simulink model "FOC_DQ0_EMR"  (R2022b)
settings: Solver=ode23s  StartTime=0.0  StopTime=50  MaxStep=1e-3
values from neighbouring files (symbols this model uses):
  battery = struct()    [FOC_DQ0_parameters.m]
  car = struct()    [FOC_DQ0_parameters.m]
  inv = struct()    [FOC_DQ0_parameters.m]
  motor = struct()    [FOC_DQ0_parameters.m]
libraries: simulink_extras x7, simulink x6, cstblocks x1
settings Model: Creator=dwegg  LastModifiedBy=dwegg
settings SolverCC: MaxConsecutiveZCs=auto  AlgebraicLoopSolver=TrustRegion
settings OptimizationCC: OptimizeBlockIOStorage=off  OptimizeDataStoreBuffers=off  BusAssignmentInplaceUpdate=off
settings DebuggingCC: UnconnectedInputMsg=warning  UnconnectedOutputMsg=warning  UnconnectedLineMsg=warning  UniqueDataStoreMsg=error  SFUnexpectedBacktrackingDiag=warning  SFNoUnconditionalDefaultTransitionDiag=warning  SFMachineParentedDataDiag=warning
settings ModelReferenceCC: EnableRefExpFcnMdlSchedulingChecks=on
settings RTWCC: GenCodeOnly=on  GenerateReport=on  BuildConfiguration=Debug  LaunchReport=on  DLArmComputeVersion=19.05
settings CodeAppCC: ForceParamTrailComments=on  MATLABSourceComments=on  EnableCustomComments=on
settings GRTTargetCC: CombineSignalStateStructs=on  SupportVariableSizeSignals=on  MultiInstanceErrorCode=Warning

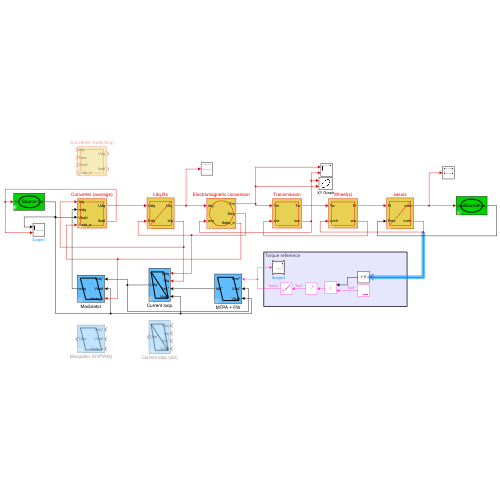
[thumbnail: Simulink's stored preview of the top-level diagram]
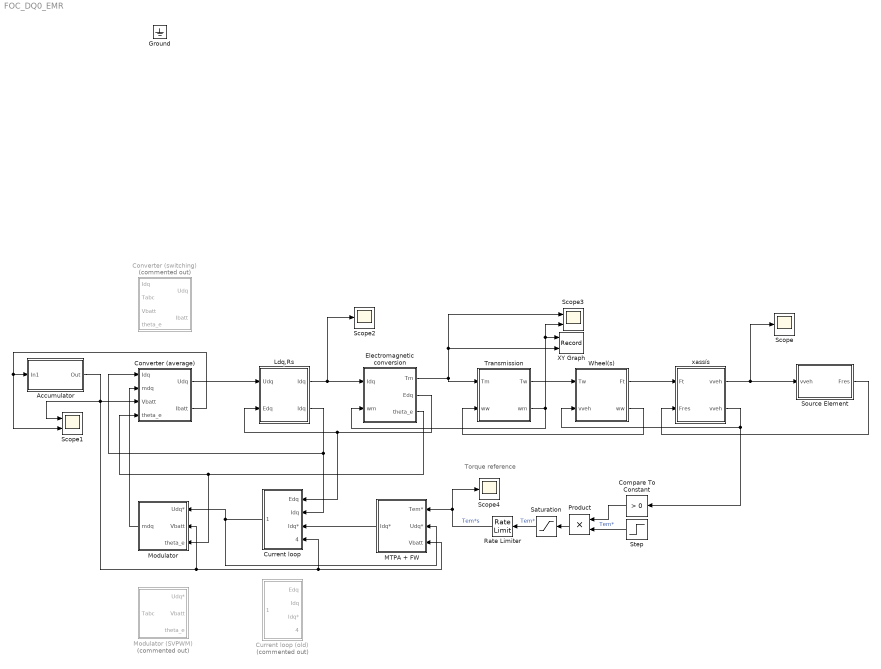
== system FOC_DQ0_EMR ==
  note: Torque reference
  Accumulator : Subsystem  AncestorBlock=simulink/REM/SE
      settings: LibrarySourceBlock=simulink/REM/SE
      mask Display:
      | plot(0,0,100,100, 1.2*[50,57.68,60.77,63.08,64.97,66.58,68,69.26,70.4, 	71.42,72.36,78.28,80,78.28,72.36,71.42,70.4, 	69.26,68,66.58,64.97,63.08,60.77,57.68,50,42.32, 	39.23,36.92,35.03,33.42,32,30.74,29.6,28.58, 	27.64,21.72,20,21.72,27.64,28.58,29.6,30.74,32, 	33.42,35.03,36.92,39.23,42.32,50]-10, 1.2*[20,21,22,23,24,25,26,27,28,29,30,40,50,60,70,71,72, 	73,74,75,76,77,78,79,80,79,78,77,76,75,74,73,72, 	71,70,60,50,40,30,29,28,27,26,25,24,23,22,21,20]-10)
      | disp('Source')
  Compare To Constant : simulink/Logic and Bit Operations/Compare To Constant  relop=>  const=0  OutDataTypeStr=boolean
  Converter (average) : Subsystem  AncestorBlock=simulink/REM/EC Elec  mask(Hacheur){}
      settings: LibrarySourceBlock=simulink/REM/EC Elec
      mask Display: plot(0,0,100,100,[10,10,90,90,10],[90,10,10,90,90])
  Converter (switching) : Subsystem  Commented=on  AncestorBlock=simulink/REM/EC Elec  mask(Hacheur){}
      settings: LibrarySourceBlock=simulink/REM/EC Elec
      mask Display: plot(0,0,100,100,[10,10,90,90,10],[90,10,10,90,90])
  Current loop : Subsystem  AncestorBlock=simulink/SMC/Asservissement Correcteur IP
      settings: LibrarySourceBlock=|
      | simulink/SMC/Asservissement
      | Correcteur IP
      mask Display: plot(0,0,100,100, [10,30,90,70,10,90],[90,10,10,90,90,10])
  Current loop (old) : Subsystem  Commented=on  AncestorBlock=simulink/SMC/Asservissement Correcteur IP
      settings: LibrarySourceBlock=|
      | simulink/SMC/Asservissement
      | Correcteur IP
      mask Display: plot(0,0,100,100, [10,30,90,70,10,90],[90,10,10,90,90,10])
  Electromagnetic conversion : Subsystem  AncestorBlock=simulink/REM/EC EM
      settings: LibrarySourceBlock=simulink/REM/EC EM
      mask Display: plot(0,0,100,100, 1.4*[50,57.68,60.77,63.08,64.97,66.58,68,69.26,70.4, 	71.42,72.36,78.28,80,78.28,72.36,71.42,70.4, 	69.26,68,66.58,64.97,63.08,60.77,57.68,50,42.32, 	39.23,36.92,35.03,33.42,32,30.74,29.6,28.58, 	27.64,21.72,20,21.72,27.64,28.58,29.6,30.74,32, 	33.42,35.03,36.92,39.23,42.32,50]-20, 1.4*[20,21,22,23,24,25,26,27,28,29,30,40,50,60,70,71,72, 	73,74,75,76,77,78,79,80,79,78,77,76,75,74,73,72, 	71,70,60,50,40,30,29,28,27,26,25,24,23,22,21,20]-20)
  Ldq,Rs : Subsystem  AncestorBlock=simulink/REM/EA  mask(CM){}
      settings: LibrarySourceBlock=simulink/REM/EA
      mask Display: plot(0,0,100,100,[10,10,90,90,10],[90,10,10,90,90], [10,90],[10,90])
  MTPA + FW : Subsystem  AncestorBlock=simulink/SMC/Inversion EC avec mesure
      settings: LibrarySourceBlock=|
      | simulink/SMC/Inversion EC
      | avec mesure
      mask Display: plot(0,0,100,100,[10,30,90,70,10],[90,10,10,90,90])
  Modulator : Subsystem  AncestorBlock=simulink/SMC/Inversion EC avec mesure
      settings: LibrarySourceBlock=|
      | simulink/SMC/Inversion EC
      | avec mesure
      mask Display: plot(0,0,100,100,[10,30,90,70,10],[90,10,10,90,90])
  Modulator (SVPWM) : Subsystem  Commented=on  AncestorBlock=simulink/SMC/Inversion EC avec mesure
      settings: LibrarySourceBlock=|
      | simulink/SMC/Inversion EC
      | avec mesure
      mask Display: plot(0,0,100,100,[10,30,90,70,10],[90,10,10,90,90])
  Product : Product
  Rate Limiter : RateLimiter  RisingSlewLimit=motor.Te_max*10  FallingSlewLimit=-motor.Te_max*10  SampleTimeMode=inherited
  Saturation : Saturate  UpperLimit=motor.Te_max*1.2  LowerLimit=-motor.Te_max*1.2
  Scope : Scope
  Scope1 : Scope  NumInputPorts=2
  Scope2 : Scope
  Scope3 : Scope  NumInputPorts=2
  Scope4 : Scope
  Source Element : Subsystem  AncestorBlock=simulink/REM/SE
      settings: LibrarySourceBlock=simulink/REM/SE
      mask Display:
      | plot(0,0,100,100, 1.2*[50,57.68,60.77,63.08,64.97,66.58,68,69.26,70.4, 	71.42,72.36,78.28,80,78.28,72.36,71.42,70.4, 	69.26,68,66.58,64.97,63.08,60.77,57.68,50,42.32, 	39.23,36.92,35.03,33.42,32,30.74,29.6,28.58, 	27.64,21.72,20,21.72,27.64,28.58,29.6,30.74,32, 	33.42,35.03,36.92,39.23,42.32,50]-10, 1.2*[20,21,22,23,24,25,26,27,28,29,30,40,50,60,70,71,72, 	73,74,75,76,77,78,79,80,79,78,77,76,75,74,73,72, 	71,70,60,50,40,30,29,28,27,26,25,24,23,22,21,20]-10)
      | disp('Source')
  Step : Step  Time=25  Before=150  After=-150  SampleTime=0
  Transmission : Subsystem  AncestorBlock=simulink/REM/EC Elec  mask(Hacheur){}
      settings: LibrarySourceBlock=simulink/REM/EC Elec
      mask Display: plot(0,0,100,100,[10,10,90,90,10],[90,10,10,90,90])
  Wheel(s) : Subsystem  AncestorBlock=simulink/REM/EC Elec  mask(Hacheur){}
      settings: LibrarySourceBlock=simulink/REM/EC Elec
      mask Display: plot(0,0,100,100,[10,10,90,90,10],[90,10,10,90,90])
  XY Graph : Record  FileSettingsInternal="{\"entries\":[{\"content\":{\"excelSettings\":{\"content\":{},\"type\":\"Streamout.ExcelSettings\"}},\"type\":\"Streamout.FileSettingStorage\",\"uuid\":\"4b251279-da9d-4be6-a887-ea3e78efb50d\"}],\"packageUris\":[\"http://schema.mathworks.com/mf0/streamout_blocks/R2020a\"],\"version\":\"1.0\"}"  Layout=[1 1]  SignalsInternal="{\"entries\":[{\"content\":{\"signals\":[{\"content\":{\"blockPath\":[\"FOC_DQ0_EMR/XY Graph\"],\"channel\":[],\"dimensions\":[1],\"domain\":\"FOC_DQ0_EMR/XY Graph\",\"lineColor\":\"#a2142f\",\"plots\":[1],\"port\":1,\"sid\":[\"\"],\"signalID\":135004,\"signalName\":\"Transmission:2\"},\"type\":\"RecordBlkView.Signal\",\"uuid\":\"7b1c68ec-b94b-4dc4-ac7b-7f2c86aeb692\"},{\"content\":{\"blockPath\":[\"FOC_DQ0_EMR/XY Graph\"],\"channel\":[],\"dimensions\":[1],\"domain\":\"FOC_DQ0_EMR/XY Graph\",\"lineColor\":\"#139fff\",\"plots\":[1],\"port\":2,\"sid\":[\"\"],\"signalID\":135008,\"signalName\":\"Electromagnetic conversion:1\"},\"type\":\"RecordBlkView.Signal\",\"uuid\":\"55ce29f7-d8dd-4043-829a-ad02527bc7f8\"}]},\"type\":\"RecordBlkView.InputSignals\",\"uuid\":\"8a0fc05b-648f-47b4-bd4d-9f4339ba604a\"}],\"packageUris\":[\"http://schema.mathworks.com/mf0/streamout_blocks/R2020a\"],\"version\":\"1.0\"}"  VisualizationBindings="{\"xyplotplugin\":{\"info\":[{\"series\":[{\"bindingParametersList\":[{\"parameter\":\"X-Axis\",\"signalID\":135004,\"signalName\":\"Transmission:2\"},{\"parameter\":\"Y-Axis\",\"signalID\":135008,\"signalName\":\"Electromagnetic conversion:1\"}],\"seriesID\":21416}],\"subplotID\":1}]}}"  CompatibilityTag=XY
  xassís : Subsystem  AncestorBlock=simulink/REM/EA  mask(CM){}
      settings: LibrarySourceBlock=simulink/REM/EA
      mask Display: plot(0,0,100,100,[10,10,90,90,10],[90,10,10,90,90], [10,90],[10,90])
  Ground : Ground  IOType=siggen
  wires:
  Accumulator/1(Out) -> Scope1/1, Converter (average)/3(Vbatt), Modulator/2(Vbatt), Current loop/4(Vbatt), MTPA + FW/3(Vbatt)
  Step/1 -> Product/2  "Tem*"
  Saturation/1 -> Rate Limiter/1  "Tem*"
  Electromagnetic conversion/2(Edq) -> Current loop/1(Edq), Ldq,Rs/2(Edq)
  Converter (average)/1(Udq) -> Ldq,Rs/1(Udq)
  Ldq,Rs/2(Idq) -> Current loop/2(Idq), Converter (average)/1(Idq)
  Converter (average)/2(Ibatt) -> Scope1/2, Accumulator/1(In1)
  Electromagnetic conversion/1(Tm) -> Transmission/1(Tm), XY Graph/2, Scope3/1
  Transmission/2(wm) -> XY Graph/1, Scope3/2, Electromagnetic conversion/2(wm)
  Transmission/1(Tw) -> Wheel(s)/1(Tw)
  Wheel(s)/2(ww) -> Transmission/2(ww)
  Current loop/1(Udq*) -> Modulator/1(Udq*), MTPA + FW/2(Udq*)
  MTPA + FW/1(Idq*) -> Current loop/3(Idq*)
  Wheel(s)/1(Ft) -> xassís/1(Ft)
  xassís/1(vveh) -> Scope/1, Source Element/1(vveh)
  Source Element/1(Fres) -> xassís/2(Fres)
  Ldq,Rs/1("Idq ") -> Scope2/1, Electromagnetic conversion/1(Idq)
  Rate Limiter/1 -> Scope4/1, MTPA + FW/1(Tem*)  "Tem*s"
  Electromagnetic conversion/3(theta_e) -> Converter (average)/4(theta_e), Modulator/3(theta_e)
  Modulator/1(mdq) -> Converter (average)/2(mdq)
  Product/1 -> Saturation/1
  Compare To Constant/1 -> Product/1
  xassís/2("vveh ") -> Compare To Constant/1, Wheel(s)/2(vveh)

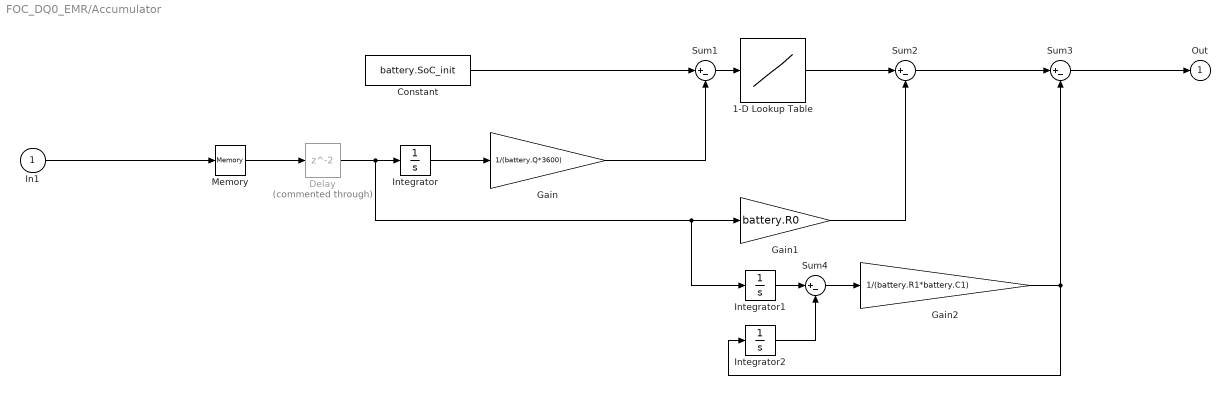
== system FOC_DQ0_EMR/Accumulator ==
  In1 : Inport
  1-D Lookup Table : Lookup_n-D  NumberOfTableDimensions=1  BreakpointsForDimension1=battery.SoC/100  Table=battery.OCV  InternalRulePriority=Speed  RndMeth=Simplest
  Constant : Constant  Value=battery.SoC_init
  Delay : Delay  Commented=through
  Gain : Gain  Gain=1/(battery.Q*3600)
  Gain1 : Gain  Gain=battery.R0
  Gain2 : Gain  Gain=1/(battery.R1*battery.C1)
  Integrator : Integrator
  Integrator1 : Integrator
  Integrator2 : Integrator
  Memory : Memory
  Sum{1..4} (4 alike) : Sum  Inputs=|+-
  Out : Outport  InitialOutput=0
  wires:
  Sum3/1 -> Out/1
  Integrator/1 -> Gain/1
  Constant/1 -> Sum1/1
  Sum1/1 -> 1-D Lookup Table/1
  Gain/1 -> Sum1/2
  1-D Lookup Table/1 -> Sum2/1
  Gain1/1 -> Sum2/2
  Sum2/1 -> Sum3/1
  Integrator1/1 -> Sum4/1
  Integrator2/1 -> Sum4/2
  Sum4/1 -> Gain2/1
  Gain2/1 -> Integrator2/1, Sum3/2
  Delay/1 -> Integrator1/1, Gain1/1, Integrator/1
  In1/1 -> Memory/1
  Memory/1 -> Delay/1

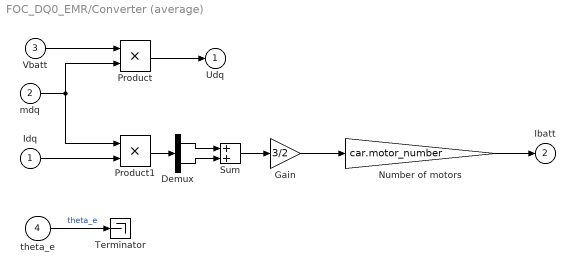
== system FOC_DQ0_EMR/Converter (average) ==
  Idq : Inport
  mdq : Inport  Port=2
  Vbatt : Inport  Port=3
  theta_e : Inport  Port=4
  Demux : Demux  Outputs=2
  Gain : Gain  Gain=3/2
  Number of motors : Gain  Gain=car.motor_number
  Product : Product
  Product1 : Product
  Sum : Sum
  Terminator : Terminator
  Udq : Outport  InitialOutput=0  VectorParamsAs1DForOutWhenUnconnected=off
  Ibatt : Outport  Port=2  InitialOutput=0  VectorParamsAs1DForOutWhenUnconnected=off
  wires:
  Vbatt/1 -> Product/1
  mdq/1 -> Product1/1, Product/2
  Product/1 -> Udq/1
  Product1/1 -> Demux/1
  Demux/1 -> Sum/1
  Demux/2 -> Sum/2
  Sum/1 -> Gain/1
  Gain/1 -> Number of motors/1
  Idq/1 -> Product1/2
  Number of motors/1 -> Ibatt/1
  theta_e/1 -> Terminator/1  "theta_e"

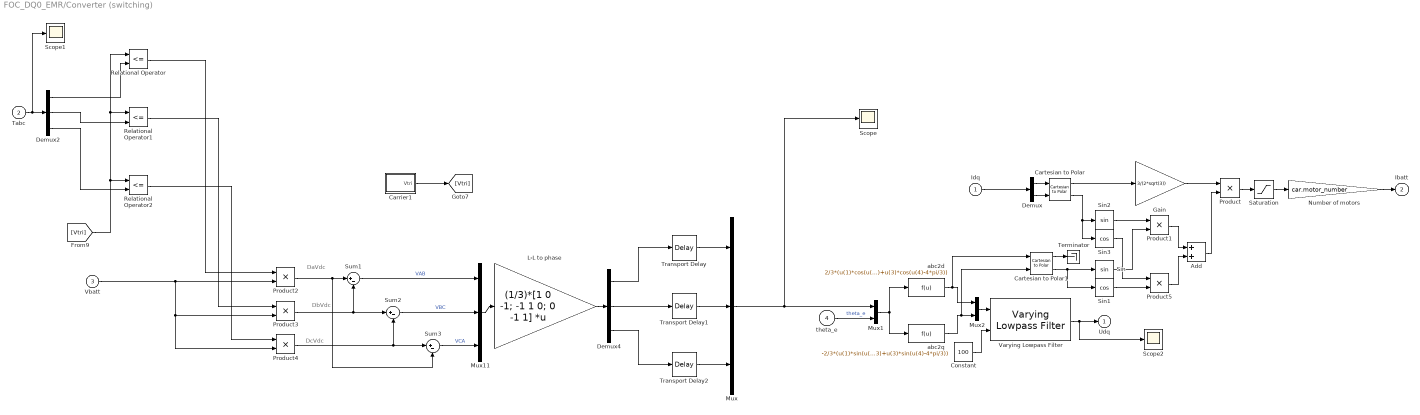
== system FOC_DQ0_EMR/Converter (switching) ==
  note: DaVdc
  note: DbVdc
  note: DcVdc
  Idq : Inport
  Tabc : Inport  Port=2
  Vbatt : Inport  Port=3
  theta_e : Inport  Port=4
  Add : Sum
  Carrier1 : Subsystem  mask{fsw=inv.fsw}
      mask prompts: fsw "switching frequency"
      mask init:
      | fsw2=fsw*2;
      | x=[0 1/4 3/4 1];
      | y=[0 -1     1    0];
      mask Display: plot([x  x+1 ],[y y])
  Cartesian to Polar : simulink_extras/Transformations/Cartesian to Polar
  Cartesian to Polar1 : simulink_extras/Transformations/Cartesian to Polar
  Constant : Constant  Value=100
  Demux : Demux  Outputs=2
  Demux2 : Demux  Outputs=3
  Demux4 : Demux  Outputs=3
  Gain : Gain  Gain=3/(2*sqrt(3))
  "L-L to phase " : Gain  Gain=(1/3)*[1 0 -1; -1 1 0; 0 -1 1]  Multiplication=Matrix(K*u)
  Mux : Mux  Inputs=3
  Mux1 : Mux  Inputs=2
  Mux11 : Mux  Inputs=3
  Mux2 : Mux  Inputs=2
  Number of motors : Gain  Gain=car.motor_number
  Product{,1..5} (6 alike) : Product
  Relational Operator : RelationalOperator  Operator=<=  OutDataTypeStr=boolean  ZeroCross=off  RndMeth=Simplest  InputSameDT=off
  Relational Operator1 : RelationalOperator  Operator=<=  OutDataTypeStr=boolean  ZeroCross=off  RndMeth=Simplest  InputSameDT=off
  Relational Operator2 : RelationalOperator  Operator=<=  OutDataTypeStr=boolean  ZeroCross=off  RndMeth=Simplest  InputSameDT=off
  Saturation : Saturate  UpperLimit=300  LowerLimit=-300
  Scope : Scope
  Scope1 : Scope
  Scope2 : Scope
  Sin : Trigonometry
  Sin1 : Trigonometry  Operator=cos
  Sin2 : Trigonometry
  Sin3 : Trigonometry  Operator=cos
  Sum1 : Sum  Inputs=|+-
  Sum2 : Sum  Inputs=|+-
  Sum3 : Sum  Inputs=|+-
  Terminator : Terminator
  Transport Delay : TransportDelay  DelayTime=inv.Tsw/2
  Transport Delay1 : TransportDelay  DelayTime=inv.Tsw/2
  Transport Delay2 : TransportDelay  DelayTime=inv.Tsw/2
  Varying Lowpass Filter : cstblocks/Linear Parameter Varying/Varying Lowpass Filter  N=1
  abc2d : Fcn  Expr=2/3*(u(1)*cos(u(4))+u(2)*cos(u(4)-2*pi/3)+u(3)*cos(u(4)-4*pi/3))
  abc2q : Fcn  Expr=-2/3*(u(1)*sin(u(4))+u(2)*sin(u(4)-2*pi/3)+u(3)*sin(u(4)-4*pi/3))
  Udq : Outport  InitialOutput=0  VectorParamsAs1DForOutWhenUnconnected=off
  Ibatt : Outport  Port=2  InitialOutput=0  VectorParamsAs1DForOutWhenUnconnected=off
  wires:
  Product/1 -> Saturation/1
  Idq/1 -> Demux/1
  Number of motors/1 -> Ibatt/1
  Demux2/1 -> Relational Operator/2
  Tabc/1 -> Scope1/1, Demux2/1
  Transport Delay2/1 -> Mux/3
  Demux4/1 -> Transport Delay/1
  Transport Delay1/1 -> Mux/2
  Relational Operator1/1 -> Product3/1
  Sum2/1 -> Mux11/2  "VBC"
  Demux4/2 -> Transport Delay1/1
  Sum1/1 -> Mux11/1  "VAB"
  Vbatt/1 -> Product4/2, Product3/2, Product2/2
  Demux4/3 -> Transport Delay2/1
  Product4/1 -> Sum3/1, Sum2/2
  Relational Operator/1 -> Product2/1
  Transport Delay/1 -> Mux/1
  "L-L to phase "/1 -> Demux4/1
  Demux2/2 -> Relational Operator1/2
  Relational Operator2/1 -> Product4/1
  Product3/1 -> Sum2/1, Sum1/2
  Carrier1/1(Vtri) -> [Vtri]
  Mux11/1 -> "L-L to phase "/1
  Demux2/3 -> Relational Operator2/2
  Sum3/1 -> Mux11/3  "VCA"
  [Vtri] -> Relational Operator1/1, Relational Operator/1, Relational Operator2/1
  Product2/1 -> Sum1/1, Sum3/2
  abc2d/1 -> Cartesian to Polar1/1, Mux2/1
  Varying Lowpass Filter/1 -> Scope2/1, Udq/1
  theta_e/1 -> Mux1/2  "theta_e"
  abc2q/1 -> Cartesian to Polar1/2, Mux2/2
  Mux/1 -> Scope/1, Mux1/1
  Mux1/1 -> abc2d/1, abc2q/1
  Demux/2 -> Cartesian to Polar/2
  Demux/1 -> Cartesian to Polar/1
  Cartesian to Polar/1 -> Gain/1
  Gain/1 -> Product/1
  Cartesian to Polar1/1 -> Terminator/1
  Cartesian to Polar1/2 -> Sin1/1, Sin/1
  Cartesian to Polar/2 -> Sin3/1, Sin2/1
  Sin2/1 -> Product1/1
  Sin/1 -> Product1/2
  Sin3/1 -> Product5/1
  Sin1/1 -> Product5/2
  Product1/1 -> Add/1
  Product5/1 -> Add/2
  Add/1 -> Product/2
  Saturation/1 -> Number of motors/1
  Mux2/1 -> Varying Lowpass Filter/1
  Constant/1 -> Varying Lowpass Filter/2

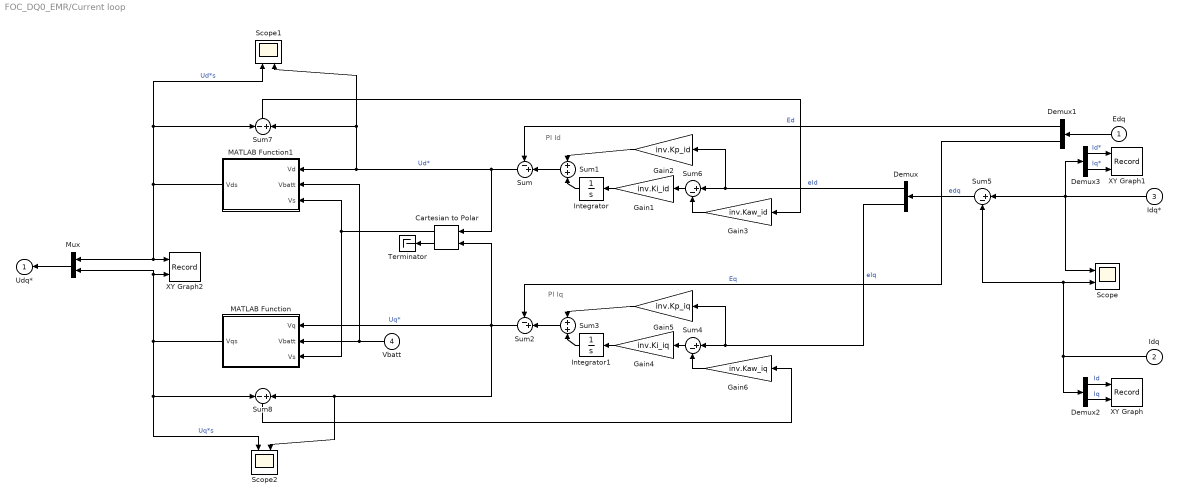
== system FOC_DQ0_EMR/Current loop ==
  note: PI Iq
  note: PI Id
  Edq : Inport
  Idq : Inport  Port=2
  Idq* : Inport  Port=3
  Vbatt : Inport  Port=4
  Cartesian to Polar : simulink_extras/Transformations/Cartesian to Polar
  Demux{,1..3} (4 alike) : Demux  Outputs=2
  Gain1 : Gain  Gain=inv.Ki_id
  Gain2 : Gain  Gain=inv.Kp_id
  Gain3 : Gain  Gain=inv.Kaw_id
  Gain4 : Gain  Gain=inv.Ki_iq
  Gain5 : Gain  Gain=inv.Kp_iq
  Gain6 : Gain  Gain=inv.Kaw_iq
  Integrator : Integrator
  Integrator1 : Integrator
  MATLAB Function : MATLAB Function  TreatAsAtomicUnit=on
  MATLAB Function1 : MATLAB Function  TreatAsAtomicUnit=on
  Mux : Mux  Inputs=2
  Scope : Scope  NumInputPorts=2
  Scope1 : Scope  NumInputPorts=2
  Scope2 : Scope  NumInputPorts=2
  Sum : Sum  Inputs=-+|
  Sum1 : Sum
  Sum2 : Sum  Inputs=-+|
  Sum3 : Sum
  Sum4 : Sum  Inputs=|+-
  Sum5 : Sum  Inputs=|+-
  Sum6 : Sum  Inputs=|+-
  Sum7 : Sum  Inputs=-+
  Sum8 : Sum  Inputs=-+
  Terminator : Terminator
  XY Graph : Record  FileSettingsInternal="{\"entries\":[{\"content\":{\"excelSettings\":{\"content\":{},\"type\":\"Streamout.ExcelSettings\"}},\"type\":\"Streamout.FileSettingStorage\",\"uuid\":\"b04a4316-fdc2-4761-b497-6a1b2ebaa3a6\"}],\"packageUris\":[\"http://schema.mathworks.com/mf0/streamout_blocks/R2020a\"],\"version\":\"1.0\"}"  Layout=[1 1]  SignalsInternal="{\"entries\":[{\"content\":{\"signals\":[{\"content\":{\"blockPath\":[\"FOC_DQ0_EMR/Current loop/XY Graph\"],\"channel\":[],\"dimensions\":[1],\"domain\":\"FOC_DQ0_EMR/Current loop/XY Graph\",\"lineColor\":\"#a2142f\",\"plots\":[1],\"port\":1,\"sid\":[\"\"],\"signalID\":135012,\"signalName\":\"Id\"},\"type\":\"RecordBlkView.Signal\",\"uuid\":\"d19068e1-5367-4519-8d0e-52a156e7d2e5\"},{\"content\":{\"blockPath\":[\"FOC_DQ0_EMR/Current loop/XY Graph\"],\"channel\":[],\"dimensions\":[1],\"domain\":\"FOC_DQ0_EMR/Current loop/XY Graph\",\"lineColor\":\"#139fff\",\"plots\":[1],\"port\":2,\"sid\":[\"\"],\"signalID\":135016,\"signalName\":\"Iq\"},\"type\":\"RecordBlkView.Signal\",\"uuid\":\"29cabb7a-c6ae-4366-a3be-e981ebbcf697\"}]},\"type\":\"RecordBlkView.InputSignals\",\"uuid\":\"9d41a52c-8fd6-4be1-80a5-12570fc5d50b\"}],\"packageUris\":[\"http://schema.mathworks.com/mf0/streamout_blocks/R2020a\"],\"version\":\"1.0\"}"  VisualizationBindings="{\"xyplotplugin\":{\"info\":[{\"series\":[{\"bindingParametersList\":[{\"parameter\":\"X-Axis\",\"signalID\":135012,\"signalName\":\"Id\"},{\"parameter\":\"Y-Axis\",\"signalID\":135016,\"signalName\":\"Iq\"}],\"seriesID\":42824}],\"subplotID\":1}]}}"  CompatibilityTag=XY
  XY Graph1 : Record  FileSettingsInternal="{\"entries\":[{\"content\":{\"excelSettings\":{\"content\":{},\"type\":\"Streamout.ExcelSettings\"}},\"type\":\"Streamout.FileSettingStorage\",\"uuid\":\"2e7905e3-53c1-4722-89d6-9879306b55d9\"}],\"packageUris\":[\"http://schema.mathworks.com/mf0/streamout_blocks/R2020a\"],\"version\":\"1.0\"}"  Layout=[1 1]  SignalsInternal="{\"entries\":[{\"content\":{\"signals\":[{\"content\":{\"blockPath\":[\"FOC_DQ0_EMR/Current loop/XY Graph1\"],\"channel\":[],\"dimensions\":[1],\"domain\":\"FOC_DQ0_EMR/Current loop/XY Graph1\",\"lineColor\":\"#a2142f\",\"plots\":[1],\"port\":1,\"sid\":[\"\"],\"signalID\":135020,\"signalName\":\"Id*\"},\"type\":\"RecordBlkView.Signal\",\"uuid\":\"31bf5c55-202d-4caa-997d-add40c8ff879\"},{\"content\":{\"blockPath\":[\"FOC_DQ0_EMR/Current loop/XY Graph1\"],\"channel\":[],\"dimensions\":[1],\"domain\":\"FOC_DQ0_EMR/Current loop/XY Graph1\",\"lineColor\":\"#139fff\",\"plots\":[1],\"port\":2,\"sid\":[\"\"],\"signalID\":135024,\"signalName\":\"Iq*\"},\"type\":\"RecordBlkView.Signal\",\"uuid\":\"1291d402-65b7-4341-aa80-d75419273496\"}]},\"type\":\"RecordBlkView.InputSignals\",\"uuid\":\"0b59ed96-63ad-4598-953c-2d5fac69a97a\"}],\"packageUris\":[\"http://schema.mathworks.com/mf0/streamout_blocks/R2020a\"],\"version\":\"1.0\"}"  VisualizationBindings="{\"xyplotplugin\":{\"info\":[{\"series\":[{\"bindingParametersList\":[{\"parameter\":\"X-Axis\",\"signalID\":135020,\"signalName\":\"Id*\"},{\"parameter\":\"Y-Axis\",\"signalID\":135024,\"signalName\":\"Iq*\"}],\"seriesID\":9552}],\"subplotID\":1}]}}"  CompatibilityTag=XY
  XY Graph2 : Record  FileSettingsInternal="{\"entries\":[{\"content\":{\"excelSettings\":{\"content\":{},\"type\":\"Streamout.ExcelSettings\"}},\"type\":\"Streamout.FileSettingStorage\",\"uuid\":\"18de3689-91cb-4cd7-80ef-e0e85249d865\"}],\"packageUris\":[\"http://schema.mathworks.com/mf0/streamout_blocks/R2020a\"],\"version\":\"1.0\"}"  Layout=[1 1]  SignalsInternal="{\"entries\":[{\"content\":{\"signals\":[{\"content\":{\"blockPath\":[\"FOC_DQ0_EMR/Current loop/XY Graph2\"],\"channel\":[],\"dimensions\":[1],\"domain\":\"FOC_DQ0_EMR/Current loop/XY Graph2\",\"lineColor\":\"#a2142f\",\"plots\":[1],\"port\":1,\"sid\":[\"\"],\"signalID\":135028,\"signalName\":\"Ud*s\"},\"type\":\"RecordBlkView.Signal\",\"uuid\":\"0d29fb7e-d738-4962-96e1-a4fd903563c3\"},{\"content\":{\"blockPath\":[\"FOC_DQ0_EMR/Current loop/XY Graph2\"],\"channel\":[],\"dimensions\":[1],\"domain\":\"FOC_DQ0_EMR/Current loop/XY Graph2\",\"lineColor\":\"#139fff\",\"plots\":[1],\"port\":2,\"sid\":[\"\"],\"signalID\":135032,\"signalName\":\"Uq*s\"},\"type\":\"RecordBlkView.Signal\",\"uuid\":\"8c3c242e-e176-4c3b-9d46-814854227cae\"}]},\"type\":\"RecordBlkView.InputSignals\",\"uuid\":\"bbd92ae3-adbd-45f7-bf59-43cc6b7ea035\"}],\"packageUris\":[\"http://schema.mathworks.com/mf0/streamout_blocks/R2020a\"],\"version\":\"1.0\"}"  VisualizationBindings="{\"xyplotplugin\":{\"info\":[{\"series\":[{\"bindingParametersList\":[{\"parameter\":\"X-Axis\",\"signalID\":135028,\"signalName\":\"Ud*s\"},{\"parameter\":\"Y-Axis\",\"signalID\":135032,\"signalName\":\"Uq*s\"}],\"seriesID\":54710}],\"subplotID\":1}]}}"  CompatibilityTag=XY
  Udq* : Outport  InitialOutput=0  VectorParamsAs1DForOutWhenUnconnected=off
  wires:
  Idq/1 -> Sum5/2, Scope/2, Demux2/1
  Mux/1 -> Udq*/1
  Sum5/1 -> Demux/1  "edq"
  Demux/1 -> Gain2/1, Sum6/1  "eId"
  Sum1/1 -> Sum/2
  Gain2/1 -> Sum1/1
  Sum6/1 -> Gain1/1
  Gain1/1 -> Integrator/1
  Integrator/1 -> Sum1/2
  Demux1/1 -> Sum/1  "Ed"
  Edq/1 -> Demux1/1
  Gain3/1 -> Sum6/2
  Gain6/1 -> Sum4/2
  Demux1/2 -> Sum2/1  "Eq"
  Integrator1/1 -> Sum3/2
  Gain4/1 -> Integrator1/1
  Sum4/1 -> Gain4/1
  Gain5/1 -> Sum3/1
  Sum3/1 -> Sum2/2
  Demux/2 -> Sum4/1, Gain5/1  "eIq"
  Sum/1 -> Sum7/2, Scope1/2, MATLAB Function1/1(Vd), Cartesian to Polar/1  "Ud*"
  Sum2/1 -> Scope2/2, Sum8/2, MATLAB Function/1(Vq), Cartesian to Polar/2  "Uq*"
  Cartesian to Polar/2 -> Terminator/1
  Cartesian to Polar/1 -> MATLAB Function1/3(Vs), MATLAB Function/3(Vs)
  Vbatt/1 -> MATLAB Function1/2(Vbatt), MATLAB Function/2(Vbatt)
  MATLAB Function1/1(Vds) -> Scope1/1, Sum7/1, XY Graph2/1, Mux/1  "Ud*s"
  MATLAB Function/1(Vqs) -> Sum8/1, Scope2/1, Mux/2, XY Graph2/2  "Uq*s"
  Sum7/1 -> Gain3/1
  Sum8/1 -> Gain6/1
  Demux2/1 -> XY Graph/1  "Id"
  Demux2/2 -> XY Graph/2  "Iq"
  Demux3/2 -> XY Graph1/2  "Iq*"
  Demux3/1 -> XY Graph1/1  "Id*"
  Idq*/1 -> Demux3/1, Scope/1, Sum5/1

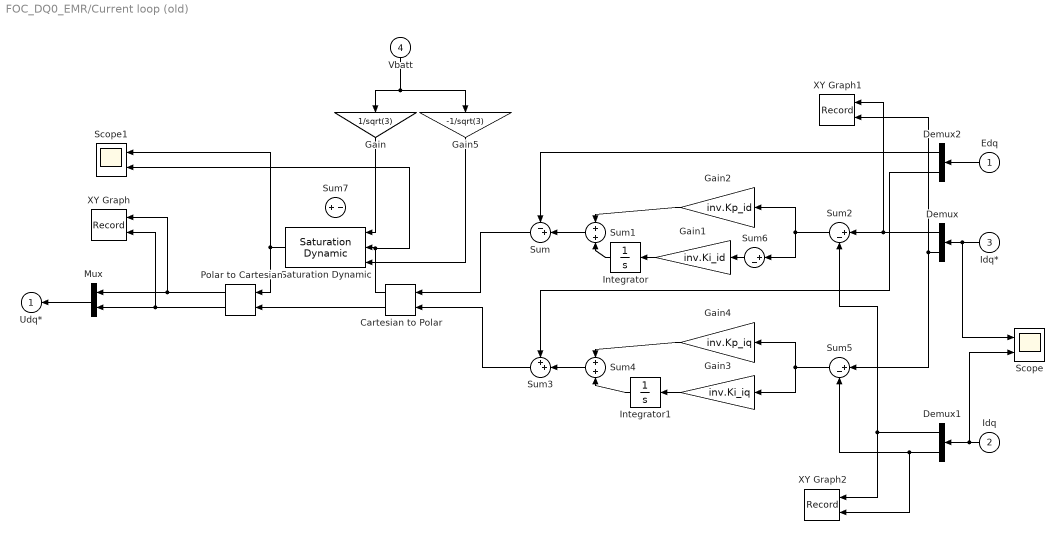
== system FOC_DQ0_EMR/Current loop (old) ==
  Edq : Inport
  Idq : Inport  Port=2
  Idq* : Inport  Port=3
  Vbatt : Inport  Port=4
  Cartesian to Polar : simulink_extras/Transformations/Cartesian to Polar
  Demux : Demux  Outputs=2
  Demux1 : Demux  Outputs=2
  Demux2 : Demux  Outputs=2
  Gain : Gain  Gain=1/sqrt(3)
  Gain1 : Gain  Gain=inv.Ki_id
  Gain2 : Gain  Gain=inv.Kp_id
  Gain3 : Gain  Gain=inv.Ki_iq
  Gain4 : Gain  Gain=inv.Kp_iq
  Gain5 : Gain  Gain=-1/sqrt(3)
  Integrator : Integrator
  Integrator1 : Integrator
  Mux : Mux  Inputs=2
  Polar to Cartesian : simulink_extras/Transformations/Polar to Cartesian
  Saturation Dynamic : simulink/Discontinuities/Saturation Dynamic  OutMin=[]  OutMax=[]  OutDataTypeStr=Inherit: Same as second input  OutDataType=fixdt(1, 16)  OutScaling=2^-10  RndMeth=Round  DoSatur=off
  Scope : Scope  NumInputPorts=2
  Scope1 : Scope  NumInputPorts=2
  Sum : Sum  Inputs=-+|
  Sum1 : Sum
  Sum2 : Sum  Inputs=|+-
  Sum3 : Sum  Inputs=++|
  Sum4 : Sum
  Sum5 : Sum  Inputs=|+-
  Sum6 : Sum  Inputs=|+-
  Sum7 : Sum  Inputs=+-
  XY Graph : Record  FileSettingsInternal="{\"entries\":[{\"content\":{\"excelSettings\":{\"content\":{},\"type\":\"Streamout.ExcelSettings\"}},\"type\":\"Streamout.FileSettingStorage\",\"uuid\":\"dc3b9b8f-4853-4122-b41a-db05675b7604\"}],\"packageUris\":[\"http://schema.mathworks.com/mf0/streamout_blocks/R2020a\"],\"version\":\"1.0\"}"  Layout=[1 1]  SignalsInternal="{\"entries\":[{\"content\":{\"signals\":[{\"content\":{\"blockPath\":[\"FOC_DQ0_EMR/Current loop (old)/XY Graph\"],\"channel\":[],\"dimensions\":[1],\"domain\":\"FOC_DQ0_EMR/Current loop (old)/XY Graph\",\"lineColor\":\"#a2142f\",\"plots\":[1],\"port\":1,\"sid\":[],\"signalID\":134954,\"signalName\":\"Polar to\\nCartesian:1\"},\"type\":\"RecordBlkView.Signal\",\"uuid\":\"3f219c77-fc2d-40fd-94f0-6f9c58e205d7\"},{\"content\":{\"blockPath\":[\"FOC_DQ0_EMR/Current loop (old)/XY Graph\"],\"channel\":[],\"dimensions\":[1],\"domain\":\"FOC_DQ0_EMR/Current loop (old)/XY Graph\",\"lineColor\":\"#139fff\",\"plots\":[1],\"port\":2,\"sid\":[],\"signalID\":134957,\"signalName\":\"Polar to\\nCartesian:2\"},\"type\":\"RecordBlkView.Signal\",\"uuid\":\"f9d73ce1-e29a-4f40-96dd-eba758a93b7a\"}]},\"type\":\"RecordBlkView.InputSignals\",\"uuid\":\"433355fb-26f9-4aec-b4d2-6e18c9961d04\"}],\"packageUris\":[\"http://schema.mathworks.com/mf0/streamout_blocks/R2020a\"],\"version\":\"1.0\"}"  VisualizationBindings="{\"xyplotplugin\":{\"info\":[{\"series\":[{\"bindingParametersList\":[{\"parameter\":\"X-Axis\",\"signalID\":134954,\"signalName\":\"Polar to\\nCartesian:1\"},{\"parameter\":\"Y-Axis\",\"signalID\":134957,\"signalName\":\"Polar to\\nCartesian:2\"}],\"seriesID\":27489}],\"subplotID\":1}]}}"  CompatibilityTag=XY
  XY Graph1 : Record  FileSettingsInternal="{\"entries\":[{\"content\":{\"excelSettings\":{\"content\":{},\"type\":\"Streamout.ExcelSettings\"}},\"type\":\"Streamout.FileSettingStorage\",\"uuid\":\"15b4ebaf-fa2f-4fe4-b46f-99fddbfef23f\"}],\"packageUris\":[\"http://schema.mathworks.com/mf0/streamout_blocks/R2020a\"],\"version\":\"1.0\"}"  Layout=[1 1]  SignalsInternal="{\"entries\":[{\"content\":{\"signals\":[{\"content\":{\"blockPath\":[\"FOC_DQ0_EMR/Current loop (old)/XY Graph1\"],\"channel\":[],\"dimensions\":[1],\"domain\":\"FOC_DQ0_EMR/Current loop (old)/XY Graph1\",\"lineColor\":\"#a2142f\",\"plots\":[1],\"port\":1,\"sid\":[],\"signalID\":134986,\"signalName\":\"Demux:1\"},\"type\":\"RecordBlkView.Signal\",\"uuid\":\"18ab1936-b0ee-4fd8-b1f9-d2df156c05ca\"},{\"content\":{\"blockPath\":[\"FOC_DQ0_EMR/Current loop (old)/XY Graph1\"],\"channel\":[],\"dimensions\":[1],\"domain\":\"FOC_DQ0_EMR/Current loop (old)/XY Graph1\",\"lineColor\":\"#139fff\",\"plots\":[1],\"port\":2,\"sid\":[],\"signalID\":134989,\"signalName\":\"Demux:2\"},\"type\":\"RecordBlkView.Signal\",\"uuid\":\"d87bdba0-8c7e-411c-993d-fcb30b4a56b5\"}]},\"type\":\"RecordBlkView.InputSignals\",\"uuid\":\"73dd423e-4535-4489-a800-02fc8de25ca2\"}],\"packageUris\":[\"http://schema.mathworks.com/mf0/streamout_blocks/R2020a\"],\"version\":\"1.0\"}"  VisualizationBindings="{\"xyplotplugin\":{\"info\":[{\"series\":[{\"bindingParametersList\":[{\"parameter\":\"X-Axis\",\"signalID\":134986,\"signalName\":\"Demux:1\"},{\"parameter\":\"Y-Axis\",\"signalID\":134989,\"signalName\":\"Demux:2\"}],\"seriesID\":15183}],\"subplotID\":1}]}}"  CompatibilityTag=XY
  XY Graph2 : Record  FileSettingsInternal="{\"entries\":[{\"content\":{\"excelSettings\":{\"content\":{},\"type\":\"Streamout.ExcelSettings\"}},\"type\":\"Streamout.FileSettingStorage\",\"uuid\":\"a683bb90-5ad5-46d6-8e59-26b01203d12d\"}],\"packageUris\":[\"http://schema.mathworks.com/mf0/streamout_blocks/R2020a\"],\"version\":\"1.0\"}"  Layout=[1 1]  SignalsInternal="{\"entries\":[{\"content\":{\"signals\":[{\"content\":{\"blockPath\":[\"FOC_DQ0_EMR/Current loop (old)/XY Graph2\"],\"channel\":[],\"dimensions\":[1],\"domain\":\"FOC_DQ0_EMR/Current loop (old)/XY Graph2\",\"lineColor\":\"#a2142f\",\"plots\":[1],\"port\":1,\"sid\":[],\"signalID\":134994,\"signalName\":\"Demux1:1\"},\"type\":\"RecordBlkView.Signal\",\"uuid\":\"2b7882d1-f238-426e-a292-a11001ebcc35\"},{\"content\":{\"blockPath\":[\"FOC_DQ0_EMR/Current loop (old)/XY Graph2\"],\"channel\":[],\"dimensions\":[1],\"domain\":\"FOC_DQ0_EMR/Current loop (old)/XY Graph2\",\"lineColor\":\"#139fff\",\"plots\":[1],\"port\":2,\"sid\":[],\"signalID\":134997,\"signalName\":\"Demux1:2\"},\"type\":\"RecordBlkView.Signal\",\"uuid\":\"277fd6a8-b415-4901-bea2-5e27c5b8d4f8\"}]},\"type\":\"RecordBlkView.InputSignals\",\"uuid\":\"c9e8b406-c351-473b-a3d6-11d74b00d187\"}],\"packageUris\":[\"http://schema.mathworks.com/mf0/streamout_blocks/R2020a\"],\"version\":\"1.0\"}"  VisualizationBindings="{\"xyplotplugin\":{\"info\":[{\"series\":[{\"bindingParametersList\":[{\"parameter\":\"X-Axis\",\"signalID\":134994,\"signalName\":\"Demux1:1\"},{\"parameter\":\"Y-Axis\",\"signalID\":134997,\"signalName\":\"Demux1:2\"}],\"seriesID\":44770}],\"subplotID\":1}]}}"  CompatibilityTag=XY
  Udq* : Outport  InitialOutput=0  VectorParamsAs1DForOutWhenUnconnected=off
  wires:
  Sum1/1 -> Sum/2
  Gain2/1 -> Sum1/1
  Integrator/1 -> Sum1/2
  Gain1/1 -> Integrator/1
  Sum2/1 -> Gain2/1, Sum6/1
  Integrator1/1 -> Sum4/2
  Gain3/1 -> Integrator1/1
  Gain4/1 -> Sum4/1
  Sum5/1 -> Gain3/1, Gain4/1
  Sum4/1 -> Sum3/2
  Idq*/1 -> Scope/1, Demux/1
  Demux/1 -> Sum2/1, XY Graph1/1
  Idq/1 -> Scope/2, Demux1/1
  Demux1/1 -> XY Graph2/1, Sum2/2
  Demux1/2 -> XY Graph2/2, Sum5/2
  Edq/1 -> Demux2/1
  Demux2/2 -> Sum3/1
  Sum/1 -> Cartesian to Polar/1
  Sum3/1 -> Cartesian to Polar/2
  Mux/1 -> Udq*/1
  Demux2/1 -> Sum/1
  Polar to Cartesian/1 -> Mux/1, XY Graph/1
  Polar to Cartesian/2 -> XY Graph/2, Mux/2
  Cartesian to Polar/1 -> Scope1/2, Saturation Dynamic/2
  Saturation Dynamic/1 -> Scope1/1, Polar to Cartesian/1
  Cartesian to Polar/2 -> Polar to Cartesian/2
  Demux/2 -> XY Graph1/2, Sum5/1
  Gain5/1 -> Saturation Dynamic/3
  Gain/1 -> Saturation Dynamic/1
  Vbatt/1 -> Gain/1, Gain5/1
  Sum6/1 -> Gain1/1

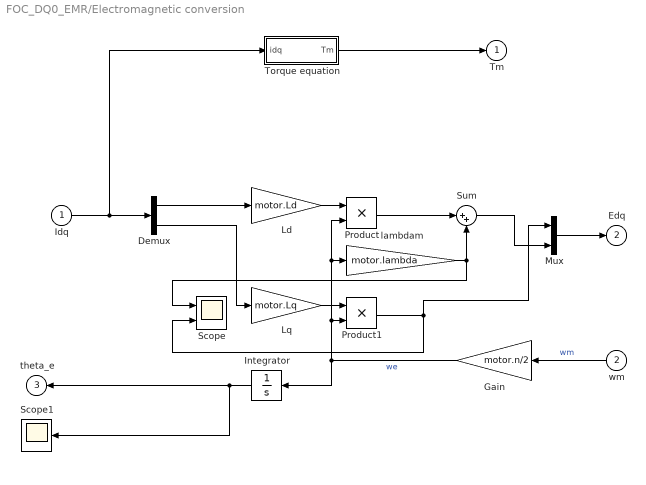
== system FOC_DQ0_EMR/Electromagnetic conversion ==
  Idq : Inport
  wm : Inport  Port=2
  Demux : Demux  Outputs=2
  Gain : Gain  Gain=motor.n/2
  Integrator : Integrator  WrapState=on  WrappedStateUpperValue=2*pi  WrappedStateLowerValue=0
  Ld : Gain  Gain=motor.Ld
  Lq : Gain  Gain=motor.Lq
  Mux : Mux  Inputs=2
  Product : Product
  Product1 : Product
  Scope : Scope  NumInputPorts=2
  Scope1 : Scope
  Sum : Sum  Inputs=|++
  Torque equation : Subsystem
  lambdam : Gain  Gain=motor.lambda
  Tm : Outport  InitialOutput=0  VectorParamsAs1DForOutWhenUnconnected=off
  Edq : Outport  Port=2  InitialOutput=0  VectorParamsAs1DForOutWhenUnconnected=off
  theta_e : Outport  Port=3  InitialOutput=0  VectorParamsAs1DForOutWhenUnconnected=off
  wires:
  Demux/1 -> Ld/1
  Demux/2 -> Lq/1
  Ld/1 -> Product/1
  wm/1 -> Gain/1  "wm"
  Lq/1 -> Product1/1
  Product/1 -> Sum/1
  lambdam/1 -> Sum/2, Scope/1
  Product1/1 -> Scope/2, Mux/1
  Mux/1 -> Edq/1
  Sum/1 -> Mux/2
  Gain/1 -> Integrator/1, Product/2, lambdam/1, Product1/2  "we"
  Idq/1 -> Torque equation/1(idq), Demux/1
  Torque equation/1(Tm) -> Tm/1
  Integrator/1 -> Scope1/1, theta_e/1

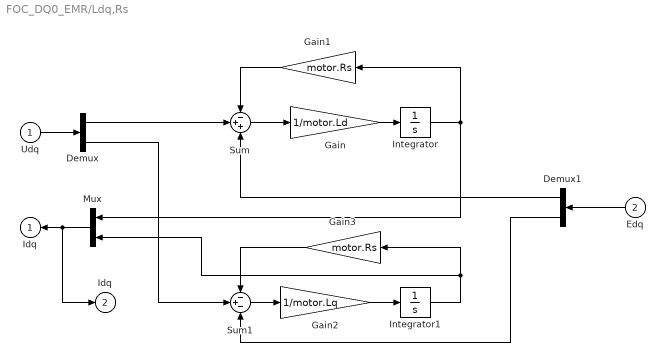
== system FOC_DQ0_EMR/Ldq,Rs ==
  Udq : Inport
  Edq : Inport  Port=2
  Demux : Demux  Outputs=2
  Demux1 : Demux  Outputs=2
  Gain : Gain  Gain=1/motor.Ld
  Gain1 : Gain  Gain=motor.Rs
  Gain2 : Gain  Gain=1/motor.Lq
  Gain3 : Gain  Gain=motor.Rs
  Integrator : Integrator
  Integrator1 : Integrator
  Mux : Mux  Inputs=2
  Sum : Sum  Inputs=-++
  Sum1 : Sum  Inputs=-+-
  "Idq " : Outport  InitialOutput=0  VectorParamsAs1DForOutWhenUnconnected=off
  Idq : Outport  Port=2  InitialOutput=0  VectorParamsAs1DForOutWhenUnconnected=off
  wires:
  Integrator/1 -> Mux/1, Gain1/1
  Gain/1 -> Integrator/1
  Sum/1 -> Gain/1
  Gain1/1 -> Sum/1
  Gain3/1 -> Sum1/1
  Gain2/1 -> Integrator1/1
  Integrator1/1 -> Gain3/1, Mux/2
  Sum1/1 -> Gain2/1
  Udq/1 -> Demux/1
  Demux/1 -> Sum/2
  Demux/2 -> Sum1/2
  Mux/1 -> Idq/1, "Idq "/1
  Edq/1 -> Demux1/1
  Demux1/1 -> Sum/3
  Demux1/2 -> Sum1/3

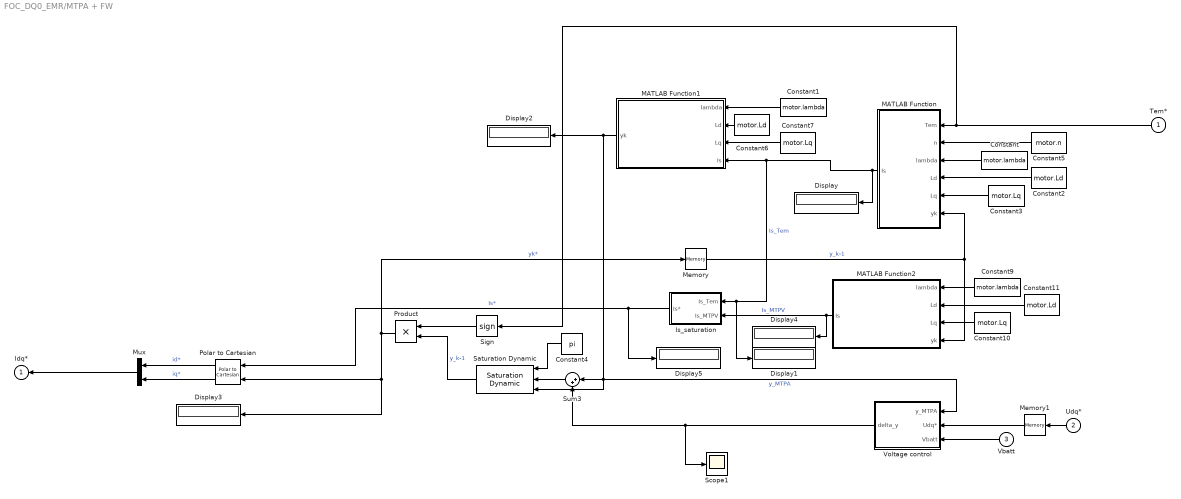
== system FOC_DQ0_EMR/MTPA + FW ==
  Tem* : Inport
  Udq* : Inport  Port=2
  Vbatt : Inport  Port=3
  Constant : Constant  Value=motor.lambda
  Constant1 : Constant  Value=motor.lambda
  Constant10 : Constant  Value=motor.Lq
  Constant11 : Constant  Value=motor.Ld
  Constant2 : Constant  Value=motor.Ld
  Constant3 : Constant  Value=motor.Lq
  Constant4 : Constant  Value=pi
  Constant5 : Constant  Value=motor.n
  Constant6 : Constant  Value=motor.Ld
  Constant7 : Constant  Value=motor.Lq
  Constant9 : Constant  Value=motor.lambda
  Display{,1..5} (6 alike) : Display
  Is_saturation : Subsystem
  MATLAB Function : MATLAB Function  TreatAsAtomicUnit=on
  MATLAB Function1 : MATLAB Function  TreatAsAtomicUnit=on
  MATLAB Function2 : MATLAB Function  TreatAsAtomicUnit=on
  Memory : Memory  InitialCondition=pi/2
  Memory1 : Memory
  Mux : Mux  Inputs=2
  Polar to Cartesian : simulink_extras/Transformations/Polar to Cartesian
  Product : Product
  Saturation Dynamic : simulink/Discontinuities/Saturation Dynamic  OutMin=[]  OutMax=[]  OutDataTypeStr=Inherit: Same as second input  OutDataType=fixdt(1, 16)  OutScaling=2^-10  DoSatur=off
  Scope1 : Scope
  Sign : Signum
  Sum3 : Sum  Inputs=|++
  Voltage control : Subsystem
  Idq* : Outport
  wires:
  Mux/1 -> Idq*/1
  Polar to Cartesian/1 -> Mux/1  "id*"
  Polar to Cartesian/2 -> Mux/2  "iq*"
  Tem*/1 -> Sign/1, MATLAB Function/1(Tem)
  MATLAB Function/1(Is) -> MATLAB Function1/4(Is), Display1/1, Is_saturation/1(Is_Tem), Display/1  "Is_Tem"
  MATLAB Function1/1(yk) -> Display2/1, Voltage control/1(y_MTPA), Saturation Dynamic/3, Sum3/1  "y_MTPA"
  Constant/1 -> MATLAB Function/3(lambda)
  Constant5/1 -> MATLAB Function/2(n)
  Constant3/1 -> MATLAB Function/5(Lq)
  Constant2/1 -> MATLAB Function/4(Ld)
  Memory/1 -> MATLAB Function/6(yk), MATLAB Function2/4(yk)  "y_k-1"
  Constant1/1 -> MATLAB Function1/1(lambda)
  Constant6/1 -> MATLAB Function1/2(Ld)
  Constant7/1 -> MATLAB Function1/3(Lq)
  Sum3/1 -> Saturation Dynamic/2
  Udq*/1 -> Memory1/1
  Vbatt/1 -> Voltage control/3(Vbatt)
  Voltage control/1(delta_y) -> Scope1/1, Sum3/2
  Constant4/1 -> Saturation Dynamic/1
  Product/1 -> Display3/1, Polar to Cartesian/2, Memory/1  "yk*"
  Constant9/1 -> MATLAB Function2/1(lambda)
  Constant10/1 -> MATLAB Function2/3(Lq)
  Constant11/1 -> MATLAB Function2/2(Ld)
  Is_saturation/1(Is*) -> Display5/1, Polar to Cartesian/1  "Is*"
  MATLAB Function2/1(Is) -> Is_saturation/2(Is_MTPV), Display4/1  "Is_MTPV"
  Memory1/1 -> Voltage control/2(Udq*)
  Sign/1 -> Product/1
  Saturation Dynamic/1 -> Product/2  "y_k-1"

== system FOC_DQ0_EMR/Modulator ==
  Udq* : Inport
  Vbatt : Inport  Port=2
  theta_e : Inport  Port=3
  Divide : Product  Inputs=*/
  Saturation : Saturate  UpperLimit=1  LowerLimit=-1
  Scope : Scope
  Terminator : Terminator
  mdq : Outport  InitialOutput=0  VectorParamsAs1DForOutWhenUnconnected=off
  wires:
  Divide/1 -> Saturation/1
  Udq*/1 -> Divide/1, Scope/1
  Vbatt/1 -> Divide/2
  Saturation/1 -> mdq/1
  theta_e/1 -> Terminator/1  "theta_e"

== system FOC_DQ0_EMR/Modulator (SVPWM) ==
  Udq* : Inport
  Vbatt : Inport  Port=2
  theta_e : Inport  Port=3
  Mux : Mux  Inputs=3
  Mux1 : Mux  Inputs=[2 1]
  SVM : MATLAB Function  TreatAsAtomicUnit=on
  alfa-axis : Fcn  Expr=u[1]*cos(u[3])-u[2]*sin(u[3])
  beta-axis : Fcn  Expr=u[1]*sin(u[3])+u[2]*cos(u[3])
  Tabc : Outport  InitialOutput=0  VectorParamsAs1DForOutWhenUnconnected=off
  wires:
  SVM/1(y) -> Tabc/1
  Mux/1 -> SVM/1(u)
  Vbatt/1 -> Mux/3
  theta_e/1 -> Mux1/2
  Udq*/1 -> Mux1/1
  Mux1/1 -> beta-axis/1, alfa-axis/1
  beta-axis/1 -> Mux/2
  alfa-axis/1 -> Mux/1

== system FOC_DQ0_EMR/Source Element ==
  vveh : Inport
  Aerodynamic drag : MATLABFcn  MATLABFcn=u^2*1.1*(1/2)*car.Af*car.Cd
  Constant : Constant  Value=0
  Constant1 : Constant  Value=0
  Rolling friction : Subsystem
  Sum : Sum  Inputs=|++
  Terminator : Terminator
  Fres : Outport  InitialOutput=0
  wires:
  vveh/1 -> Rolling friction/2(vveh), Aerodynamic drag/1
  Sum/1 -> Fres/1
  Constant/1 -> Rolling friction/1(alpha)
  Rolling friction/1(Fr) -> Terminator/1
  Aerodynamic drag/1 -> Sum/1
  Constant1/1 -> Sum/2

== system FOC_DQ0_EMR/Transmission ==
  Tm : Inport
  ww : Inport  Port=2
  Gain : Gain  Gain=car.GR
  Gain1 : Gain  Gain=car.GR
  Gain2 : Gain  Gain=60/(2*pi)
  Scope : Scope
  Tw : Outport  InitialOutput=0  VectorParamsAs1DForOutWhenUnconnected=off
  wm : Outport  Port=2  InitialOutput=0  VectorParamsAs1DForOutWhenUnconnected=off
  wires:
  Tm/1 -> Gain/1
  Gain/1 -> Tw/1
  Gain1/1 -> Gain2/1, wm/1
  ww/1 -> Gain1/1
  Gain2/1 -> Scope/1

== system FOC_DQ0_EMR/Wheel(s) ==
  Tw : Inport
  vveh : Inport  Port=2
  Gain : Gain  Gain=1/car.Rw
  Gain1 : Gain  Gain=1/car.Rw
  Number of motors : Gain  Gain=car.motor_number
  Ft : Outport  InitialOutput=0  VectorParamsAs1DForOutWhenUnconnected=off
  ww : Outport  Port=2  InitialOutput=0  VectorParamsAs1DForOutWhenUnconnected=off
  wires:
  Tw/1 -> Number of motors/1
  Gain/1 -> Ft/1
  Gain1/1 -> ww/1
  vveh/1 -> Gain1/1
  Number of motors/1 -> Gain/1

== system FOC_DQ0_EMR/xassís ==
  Ft : Inport
  Fres : Inport  Port=2
  Accel_sim : Subsystem
  Gain : Gain  Gain=1/car.Mass
  Integrator : Integrator  InitialCondition=1e-3
  Sum : Sum  Inputs=|+-
  vveh : Outport  InitialOutput=0  VectorParamsAs1DForOutWhenUnconnected=off
  "vveh " : Outport  Port=2  InitialOutput=0  VectorParamsAs1DForOutWhenUnconnected=off
  wires:
  Ft/1 -> Sum/1
  Fres/1 -> Sum/2
  Sum/1 -> Gain/1
  Gain/1 -> Integrator/1
  Integrator/1 -> vveh/1, Accel_sim/1(In1), "vveh "/1

== system FOC_DQ0_EMR/Converter (switching)/Carrier1 ==
  note: set istart time 1/fsw/4
      | set initial IC 0.5
      | to have another waveform
      |  as shown on the block
  Constant : Constant
  Constant1 : Constant  Value=2*inv.fsw
  Integrator1 : Integrator
  Product : Product  SaturateOnIntegerOverflow=on  OutDataTypeStr=Inherit: Same as first input
  Pulse Generator : DiscretePulseGenerator  PulseType=Time based  Amplitude=2  Period=1/fsw  PulseWidth=50
  Sum : Sum  Inputs=|+-  SaturateOnIntegerOverflow=on
  Vtri : Outport  InitialOutput=0  VectorParamsAs1DForOutWhenUnconnected=off
  wires:
  Pulse Generator/1 -> Sum/1
  Constant/1 -> Sum/2
  Sum/1 -> Product/1
  Constant1/1 -> Product/2
  Product/1 -> Integrator1/1
  Integrator1/1 -> Vtri/1

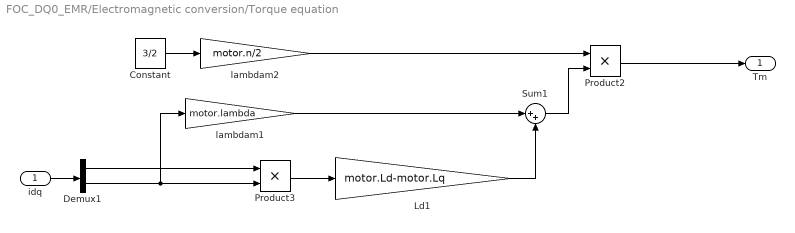
== system FOC_DQ0_EMR/Electromagnetic conversion/Torque equation ==
  idq : Inport
  Constant : Constant  Value=3/2
  Demux1 : Demux  Outputs=2
  Ld1 : Gain  Gain=motor.Ld-motor.Lq
  Product2 : Product
  Product3 : Product
  Sum1 : Sum  Inputs=|++
  lambdam1 : Gain  Gain=motor.lambda
  lambdam2 : Gain  Gain=motor.n/2
  Tm : Outport
  wires:
  lambdam1/1 -> Sum1/1
  Ld1/1 -> Sum1/2
  Product3/1 -> Ld1/1
  Sum1/1 -> Product2/2
  Constant/1 -> lambdam2/1
  Demux1/2 -> lambdam1/1, Product3/2
  lambdam2/1 -> Product2/1
  Product2/1 -> Tm/1
  Demux1/1 -> Product3/1
  idq/1 -> Demux1/1

== system FOC_DQ0_EMR/MTPA + FW/Is_saturation ==
  Is_Tem : Inport
  Is_MTPV : Inport  Port=2
  Gain : Gain  Gain=-1
  Saturation : Saturate  UpperLimit=motor.I_max  LowerLimit=0
  Saturation Dynamic1 : simulink/Discontinuities/Saturation Dynamic  OutMin=[]  OutMax=[]  OutDataTypeStr=Inherit: Same as second input  OutDataType=fixdt(1, 16)  OutScaling=2^-10  DoSatur=off
  Scope : Scope  NumInputPorts=3
  Is* : Outport
  wires:
  Saturation/1 -> Scope/2, Gain/1, Saturation Dynamic1/1  "Is_sat"
  Saturation Dynamic1/1 -> Is*/1, Scope/1  "Is*"
  Is_MTPV/1 -> Scope/3, Saturation/1
  Gain/1 -> Saturation Dynamic1/3
  Is_Tem/1 -> Saturation Dynamic1/2

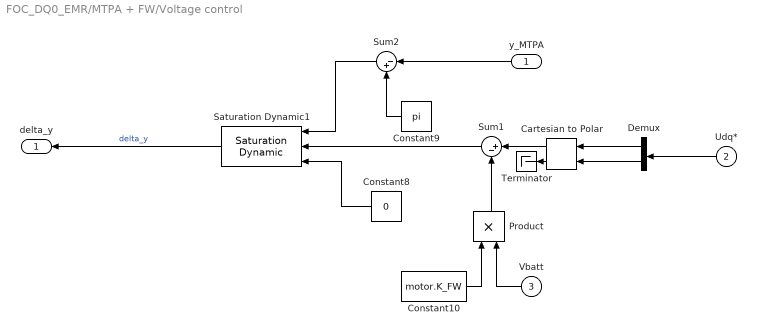
== system FOC_DQ0_EMR/MTPA + FW/Voltage control ==
  y_MTPA : Inport
  Udq* : Inport  Port=2
  Vbatt : Inport  Port=3
  Cartesian to Polar : simulink_extras/Transformations/Cartesian to Polar
  Constant10 : Constant  Value=motor.K_FW
  Constant8 : Constant  Value=0
  Constant9 : Constant  Value=pi
  Demux : Demux  Outputs=2
  Product : Product
  Saturation Dynamic1 : simulink/Discontinuities/Saturation Dynamic  OutMin=[]  OutMax=[]  OutDataTypeStr=Inherit: Same as second input  OutDataType=fixdt(1, 16)  OutScaling=2^-10  DoSatur=off
  Sum1 : Sum  Inputs=|+-
  Sum2 : Sum  Inputs=|-+
  Terminator : Terminator
  delta_y : Outport
  wires:
  Demux/1 -> Cartesian to Polar/1
  Udq*/1 -> Demux/1
  Constant8/1 -> Saturation Dynamic1/3
  Sum2/1 -> Saturation Dynamic1/1
  Vbatt/1 -> Product/2
  Product/1 -> Sum1/2
  Constant10/1 -> Product/1
  Cartesian to Polar/1 -> Sum1/1
  Saturation Dynamic1/1 -> delta_y/1  "delta_y"
  Cartesian to Polar/2 -> Terminator/1
  Demux/2 -> Cartesian to Polar/2
  Sum1/1 -> Saturation Dynamic1/2
  Constant9/1 -> Sum2/2
  y_MTPA/1 -> Sum2/1

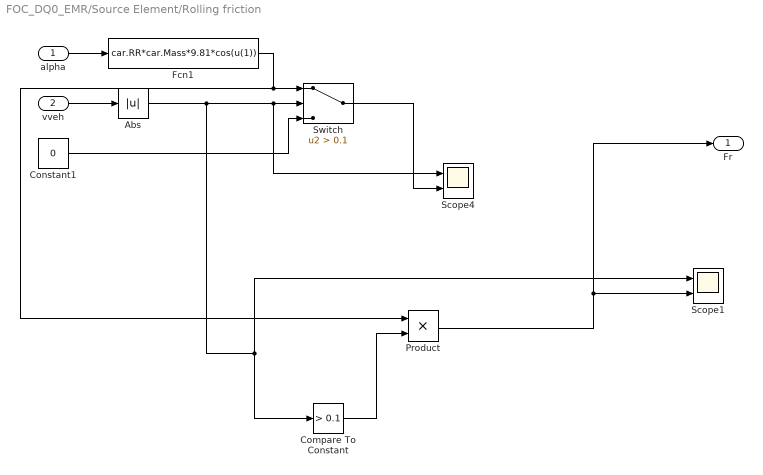
== system FOC_DQ0_EMR/Source Element/Rolling friction ==
  alpha : Inport
  vveh : Inport  Port=2
  Abs : Abs  SaturateOnIntegerOverflow=off
  Compare To Constant : simulink/Logic and Bit Operations/Compare To Constant  relop=>  const=0.1  OutDataTypeStr=boolean
  Constant1 : Constant  Value=0
  Fcn1 : Fcn  Expr=car.RR*car.Mass*9.81*cos(u(1))
  Product : Product
  Scope1 : Scope  NumInputPorts=2
  Scope4 : Scope  NumInputPorts=2
  Switch : Switch  Criteria=u2 > Threshold  Threshold=0.1  SaturateOnIntegerOverflow=off  InputSameDT=off
  Fr : Outport  VectorParamsAs1DForOutWhenUnconnected=off
  wires:
  alpha/1 -> Fcn1/1
  Switch/1 -> Scope4/2
  vveh/1 -> Abs/1
  Fcn1/1 -> Switch/1, Product/1
  Constant1/1 -> Switch/3
  Compare To Constant/1 -> Product/2
  Product/1 -> Scope1/2, Fr/1
  Abs/1 -> Scope1/1, Compare To Constant/1, Switch/2, Scope4/1

== system FOC_DQ0_EMR/xassís/Accel_sim ==
  In1 : Inport
  Constant : Constant  Value=0
  Distance [m] : Scope
  Gain2 : Gain  Gain=3.6
  If : If  IfExpression=u1 > 75
  If Action Subsystem : Subsystem  TreatAsAtomicUnit=on
  Integrator1 : Integrator
  Stop Simulation : Stop
  Terminator : Terminator
  vveh [km/h] : Scope
  wires:
  Integrator1/1 -> If/1, Distance [m]/1
  If/2 -> Terminator/1
  In1/1 -> Integrator1/1, Gain2/1
  If/1 -> If Action Subsystem/Action
  If Action Subsystem/1(Out1) -> Stop Simulation/1
  Constant/1 -> If Action Subsystem/1(In1)
  Gain2/1 -> vveh [km/h]/1

== system FOC_DQ0_EMR/xassís/Accel_sim/If Action Subsystem ==
  In1 : Inport
  Action Port : ActionPort  ActionPortLabel=if(u1 > 75)
  Out1 : Outport
  wires:
  In1/1 -> Out1/1

== matlab function FOC_DQ0_EMR/MTPA + FW/MATLAB Function1 ==
  data: lambda input size=1; Ld input size=1; Lq input size=1; yk output size=1; Is input size=1
function yk = yk_MTPA(lambda, Ld, Lq, Is)

    % Define a function that computes Te for a given Is
    compute_Is = @(yk) -lambda*cos(yk)*sec(2*yk)/(Ld-Lq);

    % Set initial guess for Is
    yk_initial_guess = pi/2; % You can adjust this value as needed

    % Use a numerical solver to find Is that satisfies the equation Te
    options = optimoptions('fsolve','Display','none','Algorithm','levenberg-marquardt');
    yk = fsolve(@(yk) compute_Is(yk)-abs(Is), yk_initial_guess, options);

end

== matlab function FOC_DQ0_EMR/MTPA + FW/MATLAB Function ==
  data: Tem input size=1; n input size=1; lambda input size=1; Ld input size=1; Lq input size=1; Is output size=1; yk input size=1
function Is = Is_Tem(Tem, n, lambda, Ld, Lq, yk)
    % Define a function that computes Te for a given Is
    compute_Te = @(Is) (3/2) * (n/2) * (Is * sin(yk) * lambda + (Ld - Lq) * Is^2 * sin(yk) * cos(yk));

    % Set initial guess for Is
    Is_initial_guess = 0; % You can adjust this value as needed

    % Use a numerical solver to find Is that satisfies the equation Te
    options = optimoptions('fsolve','Display','none','Algorithm','levenberg-marquardt');
    Is = fsolve(@(Is) compute_Te(Is) - Tem, Is_initial_guess, options);
end

== matlab function FOC_DQ0_EMR/MTPA + FW/MATLAB Function2 ==
  data: lambda input size=1; Ld input size=1; Lq input size=1; Is output size=1; yk input size=1
function Is = Is_MTPV(lambda, Ld, Lq, yk)

    Is = -lambda^2/(Ld*lambda*cos(yk)-(Lq^2/Ld)*(Ld-Lq)*sin(yk));

end

== matlab function FOC_DQ0_EMR/Modulator (SVPWM)/SVM ==
  data: u input; y output
function y = fcn(u)
% Space Vector Modulation

y                = zeros(3,1);

vsd              = u(1);  % V_alfa
vsq              = u(2);  % V_beta
Vdc              = u(3);  % DC link voltage 

% =========================================================================
% Set the voltage limits

weight           = Vdc/(sqrt(3)*sqrt(vsd*vsd+vsq*vsq));
dlimit           = abs(vsd*weight);
qlimit           = abs(vsq*weight);
if (abs(vsd)>dlimit)
    vsd          = (3*sign(vsd)*dlimit)/(2*Vdc);
else
    vsd          = (3*vsd)/(2*Vdc);
end

if(abs(vsq)>qlimit)
    vsq          = (3*sign(vsq)*qlimit)/(2*Vdc);
else
    vsq          = (3*vsq)/(2*Vdc);
end

duty_a           = 0;
duty_b           = 0;
duty_c           = 0;

% =========================================================================

if ((vsd>=0) && (vsq>=0)) 	
     if (vsq < sqrt(3)*vsd)
         % sector 0
         t1      = 0.5*(vsd-(vsq/sqrt(3)));
         t2      = vsq/sqrt(3);
         temp    = 0.5-t1-t2;
         duty_a  = 1-temp; 
         duty_b  = 1-(temp+2*t1);
         duty_c  = temp;
     else
         % sector 1
         t1      = 0.5*((vsq/sqrt(3))-vsd);
         t2      = 0.5*((vsq/sqrt(3))+vsd);
         temp    = 0.5-t1-t2;
         duty_b  = 1-temp; 
         duty_a  = 1-(temp+2*t1);
         duty_c  = temp;
     end
end

if ((vsd<0) && (vsq>0))
    if (vsq < (sqrt(3)*abs(vsd))) 
        % sector 2
        t1       = (vsq/sqrt(3));
        t2       = 0.5*(abs(vsd)-(vsq/sqrt(3)));
        temp     = 0.5-t1-t2;
        duty_b   = 1-temp; 		
        duty_c   = 1-(temp+2*t1);
        duty_a   = temp;
    else
        % sector 1
        t1       = 0.5*((vsq/sqrt(3))-vsd);
        t2       = 0.5*((vsq/sqrt(3))+vsd);
        temp     = 0.5-t1-t2;
        duty_b   = 1-temp; 	
        duty_a   = 1-(temp+2*t1);
        duty_c   = temp;
    end
end
       
if ((vsd<0) && (vsq<=0)) 	
    if (abs(vsq) <= sqrt(3)*abs(vsd)) 
        % Sector 3
        t1       = (abs(vsq)/sqrt(3));
        t2       = 0.5*(abs(vsd)-(abs(vsq)/sqrt(3)));
        temp     = 0.5-t1-t2;
        duty_c   = 1-temp; 			
        duty_b   = 1-(temp+2*t1);
        duty_a   = temp;
    else
        % Sector 4
        t1       = 0.5*((abs(vsq)/sqrt(3))-vsd);
        t2       = 0.5*((abs(vsq)/sqrt(3))+vsd);
        temp     = 0.5-t1-t2;
        duty_c   = 1-temp; 
        duty_a   = 1-(temp+2*t1);
        duty_b   = temp;
    end
end
   

if ((vsd>=0) && (vsq<0))	
    if(abs(vsq)<=vsd*sqrt(3))
        % Sector 5
        t1       = 0.5*(vsd-(abs(vsq)/sqrt(3)));
        t2       = (abs(vsq)/sqrt(3));
        temp     = 0.5-t1-t2;
        duty_a   = 1-temp; 				
        duty_c   = 1-(temp+2*t1);
        duty_b   = temp;
    else
        % Sector 4
        t1       = 0.5*((abs(vsq)/sqrt(3))-vsd);
        t2       = 0.5*((abs(vsq)/sqrt(3))+vsd);
        temp     = 0.5-t1-t2;
        duty_c   = 1-temp; 
        duty_a   = 1-(temp+2*t1);
        duty_b   = temp;
    end
end

% =========================================================================

y(1) = duty_a;
y(2) = duty_b;
y(3) = duty_c;

% =========================================================================

== matlab function FOC_DQ0_EMR/Current loop/MATLAB Function ==
  data: Vq input; Vqs output; Vbatt input; Vs input
function Vqs = voltage_limit(Vq, Vbatt, Vs)
if Vs > Vbatt / sqrt(3)
    Vqs = Vq*(Vbatt / sqrt(3))/Vs;
else
    Vqs = Vq;
end

== matlab function FOC_DQ0_EMR/Current loop/MATLAB Function1 ==
  data: Vd input; Vds output; Vbatt input; Vs input
function Vds = voltage_limit(Vd, Vbatt, Vs)
if Vs > Vbatt / sqrt(3)
    Vds = Vd*(Vbatt / sqrt(3))/Vs;
else
    Vds = Vd;
end
